simulink model "MATLAB_TEST"  (R2019b)
(part 3 of 16)

  Demux7/1 -> BUS_A429_BCMA_GenIO_2_TX/43(BCMCP_LH_antiskid_current_order)
  [V_BCM_COM_A429_AS_Curr_Order] -> Demux7/1
  Demux9/2 -> BUS_A429_BCMA_GenIO_2_TX/48(BCMCP_RH_SV_press)
  Demux9/1 -> BUS_A429_BCMA_GenIO_2_TX/47(BCMCP_LH_SV_press)
  [V_BCM_MON_A429_SP_SV_PT_PSI] -> Demux14/1
  Demux14/1 -> BUS_A429_BCMA_DFCS13_TX/21(BCMSP_LH_Brake_Pressure)
  Demux14/2 -> BUS_A429_BCMA_DFCS13_TX/22(BCMSP_RH_Brake_Pressure)
  [V_BCM_COM_A429_SV_PT_Fail] -> Demux16/1
  [V_BCM_COM_A429_SV_Fail] -> Demux15/1
  [V_BCM_COM_A429_SSM_DFCS_Label_106] -> Data Type Conversion6/1
  [V_BCM_COM_A429_SSM_DFCS_Label_107] -> Data Type Conversion7/1
  [V_BCM_COM_A429_Norm_FT_In_Progress] -> BUS_A429_BCMA_DFCS13_TX/11(BCMCP_Preland_Test)
  [V_BCM_COM_A429_Alt_FT_In_Progress] -> BUS_A429_BCMA_DFCS13_TX/12(BCMCP_Retract_Test)
  [V_BCM_COM_A429_Alt_FT_DFCS_Brkg_Req] -> BUS_A429_BCMA_DFCS13_TX/13(BCMCP_Braking_Request)
  [V_BCM_COM_A429_SSM_DFCS_Label_105] -> Data Type Conversion5/1
  [V_BCM_MON_A429_SP_RH_Brkg_Cmd_Fdbk] -> BUS_A429_BCMA_DFCS13_TX/24(BCMSP_RH_Braking_Cmd_Feedback)
  [V_BCM_MON_A429_SP_LH_Brkg_Cmd_Fdbk] -> BUS_A429_BCMA_DFCS13_TX/23(BCMSP_LH_Braking_Cmd_Feedback)
  [V_BCM_MON_A429_SP_DFCS_B_Caps_Fail] -> BUS_A429_BCMA_DFCS13_TX/26(BCMSP_DFCS_Caps_2_Fail)
  [V_BCM_MON_A429_SP_DFCS_A_Caps_Fail] -> BUS_A429_BCMA_DFCS13_TX/25(BCMSP_DFCS_Caps_1_Fail)
  [V_BCM_COM_A429_Pinprog_Fail] -> BUS_A429_BCMA_GenIO_2_TX/55(BCMCP_pinprog_fail)
  [V_BCM_COM_A429_BCM_Fail] -> BUS_A429_BCMA_DFCS13_TX/9(BCMCP_BCM_Failed)
  [V_BCM_COM_A429_BCM_Passivated] -> BUS_A429_BCMA_DFCS13_TX/10(BCMCP_BCM_Passivated)
  [V_BCM_MON_A429_SP_BCM_Failed] -> BUS_A429_BCMA_DFCS13_TX/27(BCMSP_BCM_Failed)
  [V_BCM_MON_A429_SP_BCM_Passivated] -> BUS_A429_BCMA_DFCS13_TX/28(BCMSP_BCM_Passivated)
  [V_BCM_COM_A429_LH_Brkg_Cmd_Fdbk] -> BUS_A429_BCMA_GenIO_2_TX/71(BCMCP_LH_Braking_Cmd_Feedback)
  [V_BCM_COM_A429_RH_Brkg_Cmd_Fdbk] -> BUS_A429_BCMA_GenIO_2_TX/72(BCMCP_RH_Braking_Cmd_Feedback)
  [V_BCM_COM_A429_SSM_DFCS_Label_100] -> Data Type Conversion/1
  [V_BCM_COM_A429_DFCS_B_Capsule_Fail] -> BUS_A429_BCMA_DFCS13_TX/8(BCMCP_DFCS_Caps_2_Fail)
  [V_BCM_COM_A429_DFCS_A_Capsule_Fail] -> BUS_A429_BCMA_DFCS13_TX/7(BCMCP_DFCS_Caps_1_Fail)
  Ground5/1 -> BUS_ETH_BCMA_MMS_TX/58(NLG_downlocked)
  [ETH_HYD_A_PRESS] -> BUS_ETH_BCMA_MMS_TX/54(Hydraulic_A_pressure)
  [ETH_HYD_B_PRESS] -> BUS_ETH_BCMA_MMS_TX/55(Hydraulic_B_pressure)
  [ETH_ENG1_RUNNING] -> BUS_ETH_BCMA_MMS_TX/56(Engine1_running)
  [ETH_ENG2_RUNNING] -> BUS_ETH_BCMA_MMS_TX/57(Engine2_running)
  [ETH_LMLG_Dnlk] -> BUS_ETH_BCMA_MMS_TX/59(LMLG_downlocked_raw_acquisition)
  [ETH_RMLG_Dnlk] -> BUS_ETH_BCMA_MMS_TX/60(RMLG_downlocked_raw_acquisition)
  [ETH_Lever_Up] -> BUS_ETH_BCMA_MMS_TX/61(LG_lever_up_raw_acquisition)
  Ground6/1 -> BUS_ETH_BCMA_MMS_TX/62(ESC_WonWdiscrete_raw_acquisition)
  [ETH_BCP_BCM_ALT_SW_ON_CMD] -> BUS_ETH_BCMA_MMS_TX/63(BCP_BCM_ALT_SW_ON_CMD_raw_acquisition)
  [ETH_MP_MAINT_MODE_CMD_GND] -> BUS_ETH_BCMA_MMS_TX/64(MP_MAINT_MODE_CMD_GND_raw_acquisition)
  [ETH_MAINT_MODE_CMD_28V] -> BUS_ETH_BCMA_MMS_TX/65(MP_MAINT_MODE_CMD_28V_raw_acquisition)
  [ETH_BCMA_ALT_DISP_SW] -> BUS_ETH_BCMA_MMS_TX/66(MP_BCMA_ALT_DISP_SW_raw_acquisition)
  [ETH_PBSELV_ON_POS] -> BUS_ETH_BCMA_MMS_TX/67(PBSELV_ON_POS_raw_acquisition)
  [ETH_DBCU_BRK_ORDER_FAIL] -> BUS_ETH_BCMA_MMS_TX/68(DBCU_BRK_ORDER_FAIL_raw_acquisition)
  [ETH_DISPATCH_SW_ON] -> BUS_ETH_BCMA_MMS_TX/69(DBCU_DISPATCH_SW_ON_raw_acquisition)
  [ETH_LH_DBCU_BRK_CMD_FDBK] -> BUS_ETH_BCMA_MMS_TX/70(LH_DBCU_BRK_CMD_FEEDBACK_raw_acquisition)
  [ETH_RH_DBCU_BRK_CMD_FDBK] -> BUS_ETH_BCMA_MMS_TX/71(RH_DBCU_BRK_CMD_FEEDBACK_raw_acquisition)
  [ETH_DBCU_FAILED] -> BUS_ETH_BCMA_MMS_TX/72(DBCU_FAILED_raw_acquisition)
  [ETH_ALT_MODE] -> BUS_ETH_BCMA_MMS_TX/73(DBCU_ALTERNATE_MODE_raw_acquisition)
  [ETH_Opp_BCM_DBCU_INHIB] -> BUS_ETH_BCMA_MMS_TX/74(Opposite_BCM_DBCU_INHIBITION_raw_acquisition)
  Ground7/1 -> BUS_ETH_BCMA_MMS_TX/75(BCP_PARK_OFF_SW_CMD_raw_acquisition)
  [ETH_LH_SV_Current_Order] -> BUS_ETH_BCMA_MMS_TX/76(LH_SV_current_order)
  [ETH_RH_SV_Current_Order] -> BUS_ETH_BCMA_MMS_TX/77(RH_SV_current_order)
  [ETH_SELV_High_Side_Cmd_Order] -> BUS_ETH_BCMA_MMS_TX/78(SELV_HS_order)
  [ETH_DBCU_Inhib_Order] -> BUS_ETH_BCMA_MMS_TX/79(DBCU_Inhibition_order)
  BCM_COM_PROC_P20/409(V_BCM_COM_BCM_DBCU_INHIBITION_Conf) -> Terminator13/1  "V_BCMA_COM_BCM_DBCU_INHIBITION_Conf"
  [V_BCM_COM_Adhesion_Out_W12] -> BUS_CAN_BCM_CCDL_TX/11(V_BCM_COM_Adhesion_Out_W12)
  [V_BCM_COM_Small_Slip_Trig_Out_W34] -> BUS_CAN_BCM_CCDL_TX/8(V_BCM_COM_Small_Slip_Trig_Out_W34)
  [V_BCM_COM_Target_Speed_Out_W34] -> BUS_CAN_BCM_CCDL_TX/10(V_BCM_COM_Target_Speed_Out_W34)
  [V_BCM_COM_Big_Slip_WD_Trig_Out_W12] -> BUS_CAN_BCM_CCDL_TX/5(V_BCM_COM_Big_Slip_WD_Trig_Out_W12)
  [V_BCM_COM_Big_Gamma_Trig_Out_W34] -> BUS_CAN_BCM_CCDL_TX/2(V_BCM_COM_Big_Gamma_Trig_Out_W34)
  [V_BCM_COM_Big_Slip_Trig_Out_W34] -> BUS_CAN_BCM_CCDL_TX/4(V_BCM_COM_Big_Slip_Trig_Out_W34)
  [V_BCM_COM_Big_Gamma_Trig_Out_W12] -> BUS_CAN_BCM_CCDL_TX/1(V_BCM_COM_Big_Gamma_Trig_Out_W12)
  [V_BCM_COM_Opt_Adhesion_Out_W34] -> BUS_CAN_BCM_CCDL_TX/14(V_BCM_COM_Opt_Adhesion_Out_W34)
  [V_BCM_COM_Big_Slip_WD_Trig_Out_W34] -> BUS_CAN_BCM_CCDL_TX/6(V_BCM_COM_Big_Slip_WD_Trig_Out_W34)
  [V_BCM_COM_Opt_Adhesion_Out_W12] -> BUS_CAN_BCM_CCDL_TX/13(V_BCM_COM_Opt_Adhesion_Out_W12)
  [V_BCM_COM_Small_Slip_Trig_Out_W12] -> BUS_CAN_BCM_CCDL_TX/7(V_BCM_COM_Small_Slip_Trig_Out_W12)
  [V_BCM_COM_Target_Speed_Out_W12] -> BUS_CAN_BCM_CCDL_TX/9(V_BCM_COM_Target_Speed_Out_W12)
  [V_BCM_COM_Adhesion_Out_W34] -> BUS_CAN_BCM_CCDL_TX/12(V_BCM_COM_Adhesion_Out_W34)
  [V_BCM_COM_Big_Slip_Trig_Out_W12] -> BUS_CAN_BCM_CCDL_TX/3(V_BCM_COM_Big_Slip_Trig_Out_W12)
  [BCMB_DBCU_INHIBITION] -> BCM_COM_PROC_P20/109(V_BCM_COM_BCM_DBCU_INHIBITION_Acq)
  V_BCM_COM_SELV_High_Side_Readback_Val/1 -> BCM_COM_PROC_P20/180(V_BCM_COM_SELV_High_Side_Readback_Val)
  Mux17/1 -> BCM_COM_PROC_P20/200(V_BCM_COM_SV_Current_Readback_Val)
  V_BCM_COM_SV_Current_Readback_Val/1 -> Mux17/2, Mux17/1
  Data Type Conversion/1 -> BUS_A429_BCMA_DFCS13_TX/29(LABEL_100_SSM)
  Data Type Conversion1/1 -> BUS_A429_BCMA_DFCS13_TX/30(LABEL_101_SSM)
  Data Type Conversion2/1 -> BUS_A429_BCMA_DFCS13_TX/31(LABEL_102_SSM)
  Data Type Conversion3/1 -> BUS_A429_BCMA_DFCS13_TX/32(LABEL_103_SSM)
  Data Type Conversion4/1 -> BUS_A429_BCMA_DFCS13_TX/33(LABEL_104_SSM)
  Data Type Conversion5/1 -> BUS_A429_BCMA_DFCS13_TX/34(LABEL_105_SSM)
  Data Type Conversion6/1 -> BUS_A429_BCMA_DFCS13_TX/35(LABEL_106_SSM)
  Data Type Conversion7/1 -> BUS_A429_BCMA_DFCS13_TX/36(LABEL_107_SSM)
  Data Type Conversion8/1 -> BUS_A429_BCMA_GenIO_2_TX/80(LABEL_001_SSM)
  Data Type Conversion9/1 -> BUS_A429_BCMA_GenIO_2_TX/81(LABEL_002_SSM)
  Data Type Conversion15/1 -> BUS_A429_BCMA_GenIO_2_TX/88(LABEL_012_SSM)
  Data Type Conversion10/1 -> BUS_A429_BCMA_GenIO_2_TX/82(LABEL_003_SSM)
  Data Type Conversion11/1 -> BUS_A429_BCMA_GenIO_2_TX/83(LABEL_004_SSM)
  Data Type Conversion12/1 -> BUS_A429_BCMA_GenIO_2_TX/84(LABEL_005_SSM)
  Data Type Conversion13/1 -> BUS_A429_BCMA_GenIO_2_TX/85(LABEL_006_SSM)
  Data Type Conversion14/1 -> BUS_A429_BCMA_GenIO_2_TX/86(LABEL_010_SSM)
  Data Type Conversion16/1 -> BUS_A429_BCMA_GenIO_2_TX/87(LABEL_011_SSM)
  Data Type Conversion17/1 -> BUS_A429_BCMA_GenIO_2_TX/91(LABEL_015_SSM)
  Data Type Conversion19/1 -> BUS_A429_BCMA_GenIO_2_TX/93(LABEL_017_SSM)
  Data Type Conversion18/1 -> BUS_A429_BCMA_GenIO_2_TX/92(LABEL_016_SSM)
  Data Type Conversion23/1 -> BUS_A429_BCMA_GenIO_2_TX/96(LABEL_022_SSM)
  Data Type Conversion21/1 -> BUS_A429_BCMA_GenIO_2_TX/95(LABEL_021_SSM)
  Data Type Conversion20/1 -> BUS_A429_BCMA_GenIO_2_TX/94(LABEL_020_SSM)
  Data Type Conversion24/1 -> BUS_A429_BCMA_GenIO_2_TX/89(LABEL_013_SSM)
  Data Type Conversion22/1 -> BUS_A429_BCMA_GenIO_2_TX/97(LABEL_030_SSM)
  Data Type Conversion25/1 -> BUS_A429_BCMA_GenIO_2_TX/90(LABEL_014_SSM)
  Data Type Conversion29/1 -> BUS_A429_BCMA_GenIO_2_TX/103(LABEL_036_SSM)
  Data Type Conversion26/1 -> BUS_A429_BCMA_GenIO_2_TX/100(LABEL_033_SSM)
  Data Type Conversion28/1 -> BUS_A429_BCMA_GenIO_2_TX/102(LABEL_035_SSM)
  Data Type Conversion27/1 -> BUS_A429_BCMA_GenIO_2_TX/101(LABEL_034_SSM)
  Data Type Conversion30/1 -> BUS_A429_BCMA_GenIO_2_TX/104(LABEL_037_SSM)
  Data Type Conversion32/1 -> BUS_A429_BCMA_GenIO_2_TX/105(LABEL_040_SSM)
  Data Type Conversion33/1 -> BUS_A429_BCMA_GenIO_2_TX/98(LABEL_031_SSM)
  Data Type Conversion31/1 -> BUS_A429_BCMA_GenIO_2_TX/106(LABEL_041_SSM)
  Data Type Conversion34/1 -> BUS_A429_BCMA_GenIO_2_TX/99(LABEL_032_SSM)
  Data Type Conversion35/1 -> BUS_A429_BCMA_GenIO_2_TX/107(LABEL_042_SSM)
  Data Type Conversion37/1 -> BUS_A429_BCMA_GenIO_2_TX/108(LABEL_043_SSM)
  Data Type Conversion36/1 -> BUS_A429_BCMA_GenIO_2_TX/109(LABEL_050_SSM)
  Data Type Conversion38/1 -> BUS_A429_BCMA_GenIO_2_TX/49(BCMCP_PP_channel_ID)
  HASELV_CMD_Readback/1 -> [SELV_CMD_Readback]
  RH_HASV_CURRENT_COIL1_Readback/1 -> [RH_CURRENT_COIL1_Readback]
  LH_HASV_CURRENT_COIL1_Readback/1 -> [LH_CURRENT_COIL1_Readback]
  [LH_CURRENT_COIL1_Readback] -> Mux10/1
  [RH_CURRENT_COIL1_Readback] -> Mux10/2
  Unit Delay8/1 -> BCM_COM_PROC_P5/20(V_BCM_COM_AC_State)
  DFCS1_Label206_Validity/1(Gnd_Spd_Val) -> [DFCSA_Gnd_Spd_Val]
  DFCS3_Label206_Validity/1(Gnd_Spd_Val) -> [DFCSB_Gnd_Spd_Val]
  Bus Selector4/1 -> [LNLG_Tyre_Pressure]  "<BUS_A429_LH_WRDC_BCM_LABEL_300_TyrePressure_W_1_R_LN>"
  Bus Selector4/3 -> [RMLG_Outboard_Tyre_Pressure]  "<BUS_A429_LH_WRDC_BCM_LABEL_302_TyrePressure_W_3_R_LN>"
  Bus Selector4/2 -> [LMLG_Outboard_Tyre_Pressure]  "<BUS_A429_LH_WRDC_BCM_LABEL_301_TyrePressure_W_2_R_LN>"
  Bus Selector5/1 -> [RNLG_Tyre_Pressure]  "<BUS_A429_RH_WRDC_BCM_LABEL_300_TyrePressure_W_1_R_LN>"
  Bus Selector5/2 -> [LMLG_Inboard_Tyre_Pressure]  "<BUS_A429_RH_WRDC_BCM_LABEL_301_TyrePressure_W_2_R_LN>"
  Bus Selector5/3 -> [RMLG_Inboard_Tyre_Pressure]  "<BUS_A429_RH_WRDC_BCM_LABEL_302_TyrePressure_W_3_R_LN>"
  Constant35/1 -> [CP_Inadvertent_Braking_Order_Acquisition]
  Constant36/1 -> [WheelSpeed1_Erroneous_Acquisition]
  Constant87/1 -> [WheelSpeed2_Erroneous_Acquisition]
  Constant109/1 -> [Erroneous_DBCU_Activation_On]
  Constant108/1 -> [Erroneous_DBCU_Activation_Off]
  Constant107/1 -> [CP_Erroneous_Current_RH]
  Constant114/1 -> [CP_Erroneous_Current_LH]
  Constant113/1 -> [CP_Inadvertent_Braking_Order_BSELV_DBSMA]
  Constant112/1 -> [RHPT_Erroneous_Acquisition]
  Constant111/1 -> [LHPT_Erroneous_Acquisition]
  Constant110/1 -> [WheelSpeed4_Loss]
  Constant104/1 -> [WheelSpeed3_Loss]
  Constant101/1 -> [WheelSpeed2_Loss]
  Constant100/1 -> [WheelSpeed1_Loss]
  Constant97/1 -> [WheelSpeed4_Erroneous_Acquisition]
  Constant94/1 -> [WheelSpeed3_Erroneous_Acquisition]
  Constant117/1 -> [WheelSpeed4_Erroneous_Emission]
  Constant116/1 -> [WheelSpeed3_Erroneous_Emission]
  Constant115/1 -> [WheelSpeed2_Erroneous_Emission]
  Constant118/1 -> [WheelSpeed1_Erroneous_Emission]
  Constant152/1 -> [RMLG_Inboard_Tire_Press_Unconf_Flt]
  Constant127/1 -> [RH_DBCU_BRK_CMD_FDBK_Unconf_Flt]
  Constant159/1 -> [LH_SV_PT_Conf_Flt]
  Constant148/1 -> [LMLG_Inboard_Tire_Press_Conf_Flt]
  Constant149/1 -> [LMLG_Inboard_Tire_Press_Unconf_Flt]
  Constant134/1 -> [ACCU_PT_Unconf_Flt]
  Constant157/1 -> [DFCS_B_Conf_Flt]
  Constant123/1 -> [DBCU_DISPATCH_SW_ON_Unconf_Flt]
  Constant140/1 -> [BCM_DBCU_INHIBITION_Conf_Flt]
  Constant129/1 -> [BCM_CCDL_Unconf_Flt]
  Constant162/1 -> [UTC_Time_Hours_Unconf_Flt]
  Constant165/1 -> [UTC_Time_Seconds_Conf_Flt]
  Constant160/1 -> [RH_SV_PT_Conf_Flt]
  Constant150/1 -> [RMLG_Inboard_Tire_Press_Conf_Flt]
  Constant130/1 -> [DBCU_FAILED_Unconf_Flt]
  Constant147/1 -> [LMLG_Outboard_Tire_Press_Unconf_Flt]
  Constant146/1 -> [LMLG_Outboard_Tire_Press_Conf_Flt]
  Constant133/1 -> [ACCU_PT_Conf_Flt]
  Constant153/1 -> [RMLG_Outboard_Tire_Press_Conf_Flt]
  Constant122/1 -> [DBCU_DISPATCH_SW_ON_Conf_Flt]
  Constant144/1 -> [RNLG_Tire_Press_Conf_Flt]
  Constant142/1 -> [LNLG_Tire_Press_Conf_Flt]
  Constant158/1 -> [DBCU_Conf_Flt]
  Constant141/1 -> [BCP_PARK_OFF_SW_CMD_Unconf_Flt]
  Constant145/1 -> [RNLG_Tire_Press_Unconf_Flt]
  Constant139/1 -> [BCP_PARK_OFF_SW_CMD_Conf_Flt]
  Constant138/1 -> [RH_BTS_Unconf_Flt]
  Constant136/1 -> [LH_BTS_Unconf_Flt]
  Constant126/1 -> [RH_DBCU_BRK_CMD_FDBK_Conf_Flt]
  Constant154/1 -> [RMLG_Outboard_Tire_Press_Unconf_Flt]
  Constant156/1 -> [DFCS_A_Conf_Flt]
  Constant155/1 -> [Avionics_Conf_Flt]
  Constant143/1 -> [LNLG_Tire_Press_Unconf_Flt]
  Constant163/1 -> [UTC_Time_Minutes_Conf_Flt]
  Constant137/1 -> [RH_BTS_Conf_Flt]
  Constant124/1 -> [LH_DBCU_BRK_CMD_FDBK_Conf_Flt]
  Constant125/1 -> [LH_DBCU_BRK_CMD_FDBK_Unconf_Flt]
  Constant131/1 -> [DBCU_ALT_MODE_Conf_Flt]
  Constant151/1 -> [BCM_DBCU_INHIBITION_Unconf_Flt]
  Constant119/1 -> [UTC_Time_Seconds_Unconf_Flt]
  Constant135/1 -> [LH_BTS_Conf_Flt]
  Constant164/1 -> [UTC_Time_Minutes_Unconf_Flt]
  Constant128/1 -> [DBCU_FAILED_Conf_Flt]
  Constant161/1 -> [UTC_Time_Hours_Conf_Flt]
  Constant30/1 -> [BCM_CCDL_Conf_Flt]
  Constant121/1 -> [DBCU_BRK_ORDER_FAIL_Unconf_Flt]
  Constant132/1 -> [DBCU_ALT_MODE_Unconf_Flt]
  Constant120/1 -> [DBCU_BRK_ORDER_FAIL_Conf_Flt]
  [LH_DBCU_BRK_CMD_FDBK_Conf_Flt] -> BCM_COM_PROC_P20/137(V_BCM_COM_LH_DBCU_BRK_CMD_FDBK_Conf_Flt)
  [LH_DBCU_BRK_CMD_FDBK_Unconf_Flt] -> BCM_COM_PROC_P20/138(V_BCM_COM_LH_DBCU_BRK_CMD_FDBK_Unconf_Flt)
  [Tacho_Conf_Flt] -> Selector9/1, Selector8/1
  Constant45/1 -> [CF_LH_SV_SC]
  Constant69/1 -> [CF_RH_SV_JOP]
  Constant78/1 -> [CF_SELV_OC]
  Constant67/1 -> [CF_LH_SV_OC]
  Constant85/1 -> [CF_PARK_BRK]
  Constant68/1 -> [CF_RH_SV_JCL]
  Constant63/1 -> [CF_SV_DRIFT]
  Constant65/1 -> [CF_LH_SV_JOP]
  Constant64/1 -> [CF_LH_SV_JCL]
  Constant59/1 -> [CF_BSELV_SC]
  Constant84/1 -> [CF_SELV_JCL]
  Constant77/1 -> [CF_SELV_SC]
  Constant57/1 -> [CF_RESIDUAL_PRESS]
  Constant79/1 -> [CF_SELV_JOP]
  Constant58/1 -> [CF_BSELV_OC]
  Constant71/1 -> [CF_RH_SV_OC]
  Constant61/1 -> [CF_BSELV_JOP]
  Constant70/1 -> [CF_RH_SV_SC]
  Constant60/1 -> [CF_BSELV_JCL]
  Constant62/1 -> [PPRG_Fault]
  [RH_BTS_TEMP] -> "Temperature Sensor Conversion Law mV -> °C1"/1
  "Temperature Sensor Conversion Law mV -> °C1"/1 -> BCM_COM_PROC_P20/151(V_BCM_COM_RH_BTS_TEMP_Comp)
  "Temperature Sensor Conversion Law mV -> °C"/1 -> BCM_COM_PROC_P20/148(V_BCM_COM_LH_BTS_TEMP_Comp)
  [LH_BTS_TEMP] -> "Temperature Sensor Conversion Law mV -> °C"/1
  BCM_COM_PROC_P2_5/15(V_BCM_COM_DCL_Acc) -> [V_BCM_COM_DCL_Acc]  "V_BCMA_COM_DCL_Acc"
  BCM_COM_PROC_P2_5/16(V_BCM_COM_CT_BCS_WS_First_Filter) -> Terminator38/1  "V_BCMA_COM_CT_BCS_WS_First_Filter"
  BCM_COM_PROC_P5/20(V_BCM_COM_LH_Decel_Law_Brkg_Press_Cmd) -> [V_BCM_COM_LH_Decel_Law_Brkg_Press_Cmd]  "V_BCMA_COM_LH_Decel_Law_Brkg_Press_Cmd"
  BCM_COM_PROC_P5/21(V_BCM_COM_RH_Decel_Law_Brkg_Press_Cmd) -> [V_BCM_COM_RH_Decel_Law_Brkg_Press_Cmd]  "V_BCMA_COM_RH_Decel_Law_Brkg_Press_Cmd"
  [V_BCM_COM_Global_Reference_Spd] -> Unit Delay30/1
  Unit Delay30/1 -> BCM_COM_PROC_P2_5/10(V_BCM_COM_Global_Reference_Spd)
  Unit Delay34/1 -> BCM_COM_PROC_P2_5/11(V_BCM_COM_Wheels_Global_Spun_Up_Ste)
  [V_BCM_COM_Wheels_Global_Spun_Up_Ste] -> Unit Delay34/1
  [V_BCM_COM_Wheels_Global_Spun_Up_Ste] -> Unit Delay35/1
  Unit Delay35/1 -> BCM_COM_PROC_P5/29(V_BCM_COM_Wheels_Global_Spun_Up_Ste)
  Unit Delay36/1 -> BCM_COM_PROC_P5/33(V_BCM_COM_Target_DCL)
  [V_BCM_COM_Target_DCL] -> Unit Delay36/1
  [V_BCM_COM_Global_Reference_Spd] -> Unit Delay37/1
  Unit Delay37/1 -> BCM_COM_PROC_P5/30(V_BCM_COM_Global_Reference_Spd)
  Unit Delay42/1 -> BCM_COM_PROC_P5/28(V_BCM_COM_Decel_Ctrl_Loop_Act_Cond)
  [V_BCM_COM_DCL_Acc] -> BCM_COM_PROC_P5/34(V_BCM_COM_DCL_Acc)
  [V_BCM_COM_LH_Press_Law_Brkg_Press_Cmd] -> Unit Delay38/1
  Unit Delay38/1 -> BCM_COM_PROC_P5/31(V_BCM_COM_LH_Press_Law_Brkg_Press_Cmd)
  [V_BCM_COM_RH_Press_Law_Brkg_Press_Cmd] -> Unit Delay39/1
  Unit Delay39/1 -> BCM_COM_PROC_P5/32(V_BCM_COM_RH_Press_Law_Brkg_Press_Cmd)
  [V_BCM_COM_Decel_Ctrl_Loop_Act_Cond] -> Unit Delay42/1
  [LMLG_Outboard_Tyre_Pressure] -> BCM_COM_PROC_P20/165(V_BCM_COM_LMLG_Outboard_Tire_Press_Acq)
  Logical Operator1/1 -> BCM_COM_PROC_P20/127(V_BCM_COM_DBCU_BRK_ORDER_FAIL_Acq)
  Logical Operator2/1 -> BCM_COM_PROC_P20/131(V_BCM_COM_DBCU_FAILED_Acq)
  BCM_COM_PROC_P20/411(V_BCM_COM_Decel_Ctrl_Loop_Act_Cond) -> [V_BCM_COM_Decel_Ctrl_Loop_Act_Cond]  "V_BCMA_COM_Decel_Ctrl_Loop_Act_Cond"
  COM_CAN_MON_TX/1(COM_CAN_MON) -> COM_CAN_MON/1
  [V_BCM_COM_Braking_Norm_FT_Seq] -> COM_CAN_MON_TX/1(V_BCM_COM_Braking_Norm_FT_Seq)
  [V_BCM_COM_Braking_Alt_FT_Seq] -> COM_CAN_MON_TX/2(V_BCM_COM_Braking_Alt_FT_Seq)
  [V_BCM_COM_BCM_Validity] -> COM_CAN_MON_TX/3(V_BCM_COM_BCM_Validity)
  [V_BCM_COM_Norm_Brkg_Availability] -> COM_CAN_MON_TX/4(V_BCM_COM_Norm_Brkg_Availability)
  Bus Selector3/1 -> Terminator14/1  "<V_BCMA_MON_BCM_Validity_SP>"
  Constant26/1 -> [BCM_Validity_By_SP]
  Bus Selector3/17 -> [V_BCM_MON_A429_SP_RH_Brkg_Cmd_Fdbk]  "<V_BCMA_MON_A429_SP_RH_Brkg_Cmd_Fdbk>"
  Bus Selector3/18 -> [V_BCM_MON_A429_SP_DFCS_A_Caps_Fail]  "<V_BCMA_MON_A429_SP_DFCS_A_Caps_Fail>"
  Bus Selector3/19 -> [V_BCM_MON_A429_SP_DFCS_B_Caps_Fail]  "<V_BCMA_MON_A429_SP_DFCS_B_Caps_Fail>"
  Bus Selector3/20 -> [V_BCM_MON_A429_SP_BCM_Passivated]  "<V_BCMA_MON_A429_SP_BCM_Passivated>"
  Bus Selector3/21 -> [V_BCM_MON_A429_SP_BCM_Failed]  "<V_BCMA_MON_A429_SP_BCM_Failed>"
  Bus Selector3/2 -> [V_BCM_MON_A429_SSM_DFCS_Label_121]  "<V_BCMA_MON_A429_SSM_DFCS_Label_121>"
  Bus Selector3/3 -> [V_BCM_MON_A429_SSM_DFCS_Label_122]  "<V_BCMA_MON_A429_SSM_DFCS_Label_122>"
  Bus Selector3/4 -> [V_BCM_MON_A429_SSM_DFCS_Label_123]  "<V_BCMA_MON_A429_SSM_DFCS_Label_123>"
  Bus Selector3/5 -> [V_BCM_MON_A429_SSM_DFCS_Label_124]  "<V_BCMA_MON_A429_SSM_DFCS_Label_124>"
  Bus Selector3/6 -> [V_BCM_MON_A429_SSM_DFCS_Label_125]  "<V_BCMA_MON_A429_SSM_DFCS_Label_125>"
  Bus Selector3/7 -> [V_BCM_MON_A429_SSM_DFCS_Label_126]  "<V_BCMA_MON_A429_SSM_DFCS_Label_126>"
  Bus Selector3/8 -> [V_BCM_MON_A429_SSM_DFCS_Label_127]  "<V_BCMA_MON_A429_SSM_DFCS_Label_127>"
  Bus Selector3/9 -> [V_BCM_MON_A429_SSM_DFCS_Label_130]  "<V_BCMA_MON_A429_SSM_DFCS_Label_130>"
  Bus Selector3/10 -> [V_BCM_MON_A429_SSM_DFCS_Label_131]  "<V_BCMA_MON_A429_SSM_DFCS_Label_131>"
  Bus Selector3/11 -> [V_BCM_MON_A429_SSM_DFCS_Label_150]  "<V_BCMA_MON_A429_SSM_DFCS_Label_150>"
  Bus Selector3/12 -> [V_BCM_MON_A429_SSM_DFCS_Label_151]  "<V_BCMA_MON_A429_SSM_DFCS_Label_151>"
  Bus Selector3/13 -> [V_BCM_MON_A429_SP_Wheel_Speed_W12]  "<V_BCMA_MON_A429_SP_Wheel_Speed_W12>"
  Bus Selector3/14 -> [V_BCM_MON_A429_SP_Wheel_Speed_W34]  "<V_BCMA_MON_A429_SP_Wheel_Speed_W34>"
  Bus Selector3/15 -> [V_BCM_MON_A429_SP_SV_PT_PSI]  "<V_BCMA_MON_A429_SP_SV_PT_PSI>"
  Bus Selector3/16 -> [V_BCM_MON_A429_SP_LH_Brkg_Cmd_Fdbk]  "<V_BCMA_MON_A429_SP_LH_Brkg_Cmd_Fdbk>"
  [V_BCM_MON_A429_SSM_DFCS_Label_121] -> Data Type Conversion39/1
  Data Type Conversion47/1 -> BUS_A429_BCMA_DFCS13_TX/45(LABEL_131_SSM)
  Data Type Conversion48/1 -> BUS_A429_BCMA_DFCS13_TX/46(LABEL_150_SSM)
  Data Type Conversion39/1 -> BUS_A429_BCMA_DFCS13_TX/37(LABEL_121_SSM)
  Data Type Conversion40/1 -> BUS_A429_BCMA_DFCS13_TX/38(LABEL_122_SSM)
  Data Type Conversion41/1 -> BUS_A429_BCMA_DFCS13_TX/39(LABEL_123_SSM)
  Data Type Conversion42/1 -> BUS_A429_BCMA_DFCS13_TX/40(LABEL_124_SSM)
  Data Type Conversion43/1 -> BUS_A429_BCMA_DFCS13_TX/41(LABEL_125_SSM)
  Data Type Conversion44/1 -> BUS_A429_BCMA_DFCS13_TX/42(LABEL_126_SSM)
  Data Type Conversion45/1 -> BUS_A429_BCMA_DFCS13_TX/43(LABEL_127_SSM)
  Data Type Conversion46/1 -> BUS_A429_BCMA_DFCS13_TX/44(LABEL_130_SSM)
  [V_BCM_MON_A429_SSM_DFCS_Label_122] -> Data Type Conversion40/1
  [V_BCM_MON_A429_SSM_DFCS_Label_123] -> Data Type Conversion41/1
  [V_BCM_MON_A429_SSM_DFCS_Label_124] -> Data Type Conversion42/1
  [V_BCM_MON_A429_SSM_DFCS_Label_125] -> Data Type Conversion43/1
  [V_BCM_MON_A429_SSM_DFCS_Label_126] -> Data Type Conversion44/1
  [V_BCM_MON_A429_SSM_DFCS_Label_127] -> Data Type Conversion45/1
  [V_BCM_MON_A429_SSM_DFCS_Label_130] -> Data Type Conversion46/1
  [V_BCM_MON_A429_SSM_DFCS_Label_131] -> Data Type Conversion47/1
  [V_BCM_MON_A429_SSM_DFCS_Label_150] -> Data Type Conversion48/1
  [V_BCM_MON_A429_SSM_DFCS_Label_151] -> Data Type Conversion49/1
  Data Type Conversion49/1 -> BUS_A429_BCMA_DFCS13_TX/47(LABEL_151_SSM)
  BCM_COM_PROC_P20/410(V_BCM_COM_Target_DCL) -> [V_BCM_COM_Target_DCL]  "V_BCMA_COM_Target_DCL"
  DFCS1_Label204_Validity/7(ALT_Mode_1_Val) -> [DFCSA_ALT_Mode_1_Val]
  DFCS1_Label204_Validity/8(ALT_Mode_2_Val) -> [DFCSA_ALT_Mode_2_Val]
  DFCS3_Label204_Validity/7(ALT_Mode_1_Val) -> [DFCSB_ALT_Mode_1_Val]
  DFCS3_Label204_Validity/8(ALT_Mode_2_Val) -> [DFCSB_ALT_Mode_2_Val]
  Constant27/1 -> Terminator18/1
